simulink model "converting_celcius_fahrenite"  (R2020a)
settings: Solver=VariableStepAuto  StartTime=0.0  StopTime=10.0  RelTol=1e-3
settings Model: Creator=Ganesh  LastModifiedBy=Ganesh

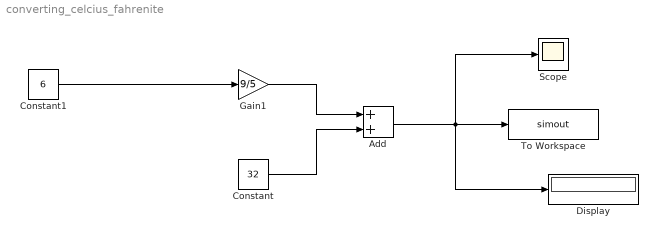
== system converting_celcius_fahrenite ==
  Add : Sum
  Constant : Constant  Value=32
  Constant1 : Constant  Value=6
  Display : Display
  Gain1 : Gain  Gain=9/5
  Scope : Scope
  To Workspace : ToWorkspace  VariableName=simout  SaveFormat=Timeseries  SampleTime=-1
  wires:
  Add/1 -> Display/1, Scope/1, To Workspace/1
  Constant/1 -> Add/2
  Gain1/1 -> Add/1
  Constant1/1 -> Gain1/1
